simulink model "TDPBehaviourSim2"  (R2020b)
settings: Solver=FixedStepAuto  StartTime=0.0  StopTime=200  FixedStep=sampleTime  RelTol=1e-3  EnableMultiTasking=on
values from neighbouring files (symbols this model uses):
  angThresh = pi/16    (= 0.196349540849)    [GameParameters.m]
  attackerKickSpeed = 0.3    [GameParameters.m]
  AwayFormation1 = [9.5 4 pi ... (first row only)    [FormationPoses.m]    (also in GameParameters.m)
  ballAngleNoise = pi/24    (= 0.1308996939)    [GameParameters.m]
  ballThresh = playerRadius + 0.03    (= 0.11)    [GameParameters.m]
  ballVelNoise = 0.05    [GameParameters.m]
  distThresh = 0.1    [GameParameters.m]
  fieldCenter = [mean(fieldLimitsX) mean(fieldLimitsY)]    [GameParameters.m]
  fieldLimitsX = [1 10]    [GameParameters.m]
  fieldLimitsY = [1 7]    [GameParameters.m]
  goalPosts = [1  2.7 2 ... (first row only)    [GameParameters.m]
  HomeFormation1 = [1.5 4 0 ... (first row only)    [FormationPoses.m]    (also in GameParameters.m)
  maxSpeed = 0.1    [GameParameters.m]
  maxTurnSpeed = 0.05    [GameParameters.m]
  playerIdx = (0:8)    [GameParameters.m]
  playerRadius = 0.08    [GameParameters.m]
  sampleTime = 0.1    [GameParameters.m]
undefined symbols (not defined in the file or in its folder): DiscIntNeverNeededParam
libraries: mobileRoboticsLib x33, soccerRobotLib x16
(part 2 of 2)

== stateflow chart TDPBehaviourSim2/Home Team/Chart3 ==
  state BallInteraction [parallel]
    en,du:
    toBall = [gkObjSeen,gkObjDist,gkObjAng;
    defObjSeen,defObjDist,defObjAng;
    midObjSeen,midObjDist,midObjAng;
    stkObjSeen,stkObjDist,stkObjAng]
    settings: executionOrder=2
  state MoveTeam [parallel]
    en,du:
    settings: executionOrder=1
    state Attack
      en,du:
      state GoalKeeper [parallel]
        en,du:
        [gkObjSeen,gkObjDist,gkObjAng]=detectObj(gk.objectDetections,1)
        settings: executionOrder=1
      state Defender [parallel]
        en,du:
        [defObjSeen,defObjDist,defObjAng]=detectObj(def.objectDetections,1);
        settings: executionOrder=2
      state MidFielder [parallel]
        en,du:
        [midObjSeen,midObjDist,midObjAng]=detectObj(mid.objectDetections,1);
        settings: executionOrder=3
      state Striker [parallel]
        en,du:
        [stkObjSeen,stkObjDist,stkObjAng]=detectObj(stk.objectDetections,1)
        settings: executionOrder=4
        state InPossession
          en,du:
          nextVel.stk = goToPose([8,4,pi],stk.position);
        state TeammateInPossession
          en,du:
        (default) -> (junction 231)
        (junction 231) -> InPossession [order 1] : [homeTeam.possession(1)==1 &&...
            | homeTeam.possession(2)==playerIdx(5)]
        (junction 231) -> (junction 236) [order 2]
        InPossession -> TeammateInPossession : [homeTeam.possession(1)==1 &&...
            | homeTeam.possession(2)~=playerIdx(5)]
        TeammateInPossession -> InPossession : [homeTeam.possession(1)==1 &&...
            | homeTeam.possession(2)==playerIdx(5)]
        (junction 236) -> TeammateInPossession
    state Defend
      en,du:
      state GoalKeeper [parallel]
        en,du:
        [gkObjSeen,gkObjDist,gkObjAng]=detectObj(gk.objectDetections,1)
        settings: executionOrder=3
      state Defender [parallel]
        en,du:
        [defObjSeen,defObjDist,defObjAng]=detectObj(def.objectDetections,1);
        settings: executionOrder=4
      state MidFielder [parallel]
        en,du:
        [midObjSeen,midObjDist,midObjAng]=detectObj(mid.objectDetections,1);
        settings: executionOrder=1
      state Striker [parallel]
        en,du:
        [stkObjSeen,stkObjDist,stkObjAng]=detectObj(stk.objectDetections,1)
        settings: executionOrder=2
    state CaptureBall
      en,du:
      state GoalKeeper [parallel]
        en,du:
        [gkObjSeen,gkObjDist,gkObjAng]=detectObj(gk.objectDetections,1)
        settings: executionOrder=3
      state Defender [parallel]
        en,du:
        [defObjSeen,defObjDist,defObjAng]=detectObj(def.objectDetections,1);
        settings: executionOrder=4
      state MidFielder [parallel]
        en,du:
        [midObjSeen,midObjDist,midObjAng]=detectObj(mid.objectDetections,1);
        settings: executionOrder=1
      state Striker [parallel]
        en,du:
        [stkObjSeen,stkObjDist,stkObjAng]=detectObj(stk.objectDetections,1);
        settings: executionOrder=2
        state StayStationery
          en,du:
          [stkObjSeen,stkObjDist,stkObjAng]=detectObj(stk.objectDetections,1);
          nextVel.stk = [0;0;-0.02];
        state GoToBall
          en,du:
          nextVel.stk=trackDetection(stkObjDist,stkObjAng);
        (default) -> StayStationery
        StayStationery -> GoToBall : [stkObjSeen&&stkObjDist<2.5&&stkObjAng<pi/8]
    (default) -> (junction 172)
    (junction 225) -> Attack : [homeTeam.possessingTeam==1]
    (junction 226) -> (junction 225)
    (junction 172) -> Attack [order 1] : [homeTeam.possessingTeam==1]
    (junction 172) -> (junction 173) [order 2]
    Attack -> Defend : [homeTeam.possessingTeam==2]
    Defend -> Attack [order 1] : [homeTeam.possessingTeam==1]
    (junction 173) -> Defend [order 1] : [homeTeam.possessingTeam==2]
    (junction 173) -> (junction 191) [order 2]
    CaptureBall -> Defend [order 1] : [homeTeam.possessingTeam==2]
    Defend -> CaptureBall [order 2] : [homeTeam.possessingTeam==0]
    CaptureBall -> (junction 226) [order 2]
    (junction 191) -> CaptureBall
  state [vel,done] = goToPose(goal,position) [function]
    note: Tracks a position. Once reached, the robot will turn in place until a reference angle is met.
    (default) -> (junction 9) : {
        | vel = [0;0;0];
        | [goalDist,goalAng] = calcBearing(goal(1:2),position);
        | trackAng = angdiff(position(3),goal(3));
        | }
    (junction 9) -> (junction 10) [order 1] : % Track the position if outside the distance threshold
        | [goalDist > distThresh]
    (junction 9) -> (junction 11) [order 2] : % Else, turn in place until the angular reference is met
    (junction 10) -> (junction 18) : {vel = trackDetection(goalDist,goalAng);}
    (junction 11) -> (junction 12) [order 1] : [trackAng > angThresh]
    (junction 12) -> (junction 17) : {vel(3) = 0.01;}
    (junction 11) -> (junction 13) [order 2]
    (junction 13) -> (junction 14) [order 1] : [trackAng < -angThresh]
    (junction 14) -> (junction 16) : {vel(3) = -0.01;}
    (junction 13) -> (junction 15) [order 2]
    (junction 16) -> (junction 15)
    (junction 17) -> (junction 16)
    (junction 18) -> (junction 17)
    (junction 15) -> (junction 19) : {done = (goalDist <= distThresh) && (abs(trackAng) <= angThresh);}
  state [dist,ang] = calcBearing(goal,position) [function]
    (default) -> (junction 39) : % Calculate distance and angle to location
        | {
        | err = goal(1:2) - [position(1) position(2)];
        | dist = norm(err);
        | ang = angdiff(position(3),atan2(err(2),err(1)));
        | }
  state [vel,done] = turnToPoint(goal) [function]
    note: Tracks a position. Once reached, the robot will turn in place until a reference angle is met.
    (default) -> (junction 82) : % Turn in place until the angular reference is met
        | {
        | done = false;
        | vel = [0;0;0];
        | [goalDist,goalAng] = calcBearing(goal(1:2));
        | }
    (junction 82) -> (junction 83) [order 1] : [goalAng > angThresh]
    (junction 82) -> (junction 84) [order 2]
    (junction 83) -> (junction 88) : {vel(3) = 0.02;}
    (junction 84) -> (junction 85) [order 1] : [goalAng < -angThresh]
    (junction 85) -> (junction 87) : {vel(3) = -0.02;}
    (junction 84) -> (junction 86) [order 2] : {done = true;}
    (junction 87) -> (junction 86)
    (junction 88) -> (junction 87)
  state vel = trackDetection(dist,ang) [function]
    note: Uses range and bearing to track an object
    (default) -> (junction 46) : {
        | vel = [0;0;0];
        | }
    (junction 46) -> (junction 45) [order 1] : % Turn in place
        | % if no detection
        | [dist < 0]
    (junction 45) -> (junction 55) : {vel(3) = 1;}
    (junction 46) -> (junction 47) [order 2]
    (junction 47) -> (junction 48) [order 1] : % Forward speed
        | [dist > distThresh]
    (junction 47) -> (junction 49) [order 2]
    (junction 48) -> (junction 50) : {vel(1) = maxSpeed;}
    (junction 50) -> (junction 49)
    (junction 49) -> (junction 51)
    (junction 51) -> (junction 52) [order 1] : % Turning speed
        | [ang > angThresh]
    (junction 51) -> (junction 53) [order 2]
    (junction 52) -> (junction 58) : {vel(3) = maxTurnSpeed;}
    (junction 53) -> (junction 54) [order 1] : [ang < -angThresh]
    (junction 53) -> (junction 56) [order 2]
    (junction 54) -> (junction 57) : {vel(3) = -maxSpeed;}
    (junction 55) -> (junction 56)
    (junction 57) -> (junction 56)
    (junction 58) -> (junction 57)
  data: vel function_output; done function_output; goal function_input; position function_input; goal function_input; dist function_output; ang function_output; position function_input; goal function_input; vel function_output; done function_output; dist function_input; ang function_input; vel function_output; detections function_input; obj function_input; objSeen function_output; objRange function_output; objAngle function_output; homeTeam input Bus: gameSituationBus; gk input Bus: PlayerStateBus; def input Bus: PlayerStateBus; defObjSeen local boolean =false; defObjAng local =0; defObjDist local =-1; mid input Bus: PlayerStateBus; midObjSeen local boolean =false; midObjDist local =-1; midObjAng local =0; stk input Bus: PlayerStateBus; stkObjAng local =0; stkObjDist local =-1; stkObjSeen local boolean =false; toBall output; nextVel output Bus: nextVel; gkObjAng local =0; gkObjDist local =-1; gkObjSeen local boolean =false; maxSpeed parameter; maxTurnSpeed parameter; distThresh parameter; angThresh parameter; playerIdx parameter; stkPos local size=[3]
  function [objSeen, objRange,objAngle] = detectObj(detections,obj):
    | function [objSeen, objRange,objAngle] = detectObj(detections,obj)
    | % Accepts a set of object detections and searches for a ball
    | %
    | % Copyright 2019 The MathWorks, Inc.
    | objSeen = 0;
    | objRange = -1;
    | objAngle =  0;
    | 
    | objSeen = ~isempty(find(detections(:,3)==obj,1));
    | 
    | for idx = 1:size(detections,1)
    |     if detections(idx,3) == obj
    |         objRange = detections(idx,1);
    |         objAngle = detections(idx,2);
    |     end
    | end
    | 
    | end
